simulink model "gm_combinedTxRx_AXIMM"  (R2017b)
settings: Solver=FixedStepDiscrete  StartTime=0.0  StopTime=10.0  RelTol=1e-3
InitFcn:
  | modelSettings
undefined symbols (not defined in the file or in its folder): coeff, filt, j, RadioSampleRate, VibertiTracebackLength, xPreambleSeq
libraries: hdlmdlgenlib x24, simulink x20, dsphdlfiltering x20, hdlsllib x10, dspsigops x5, commseqgen3 x4, commdigbbndpm3 x3, commcrc2 x2, commcnvcod2 x2, commsource2 x1, dspstat3 x1, dspmlti4 x1
(part 5 of 6)

== system gm_combinedTxRx_AXIMM/Combined TX and RX/Receiver HDL/Frame Recover/Gardner Timing Recovery/InterpControl_Blocks1/Calculate New mu ==
  note: Good at fixd(0,16,12)
  W : Inport  SampleTime=1e-06
  NCOCounter : Inport  Port=2  SampleTime=1e-06
  Math Reciprocal : Math  Operator=reciprocal  OutDataTypeStr=fixdt(1,16,12)  RndMeth=Zero  SaturateOnIntegerOverflow=on
  Product : Product  OutDataTypeStr=fixdt(0,15,14)
  mu : Outport  InitialOutput=0
  wires:
  W/1 -> Math Reciprocal/1
  NCOCounter/1 -> Product/2
  Math Reciprocal/1 -> Product/1
  Product/1 -> mu/1

== system gm_combinedTxRx_AXIMM/Combined TX and RX/Receiver HDL/Frame Recover/Gardner Timing Recovery/InterpControl_Blocks1/Mod 1 ==
  In1 : Inport  SampleTime=1e-06
  Add : Sum
  Compare To Constant : simulink/Logic and Bit Operations/Compare To Constant  relop=<  const=1  OutDataTypeStr=boolean
  Compare To Constant1 : simulink/Logic and Bit Operations/Compare To Constant  relop=>=  const=0  OutDataTypeStr=boolean
  Constant : Constant  OutDataTypeStr=fixdt(0,1,0)  SampleTime=-1
  Constant1 : Constant  OutDataTypeStr=fixdt(0,1,0)  SampleTime=-1
  Logical Operator : Logic  AllPortsSameDT=off  OutDataTypeStr=boolean
  Subtract : Sum  Inputs=+-
  Switch : Switch  Criteria=u2 > Threshold
  Switch1 : Switch
  Out1 : Outport  InitialOutput=0
  wires:
  In1/1 -> Switch1/2, Switch/1, Subtract/1, Compare To Constant1/1, Compare To Constant/1, Add/1
  Add/1 -> Switch1/3
  Compare To Constant/1 -> Logical Operator/2
  Compare To Constant1/1 -> Logical Operator/1
  Constant/1 -> Subtract/2
  Constant1/1 -> Add/2
  Logical Operator/1 -> Switch/2
  Subtract/1 -> Switch1/1
  Switch/1 -> Out1/1
  Switch1/1 -> Switch/3

== system gm_combinedTxRx_AXIMM/Combined TX and RX/Receiver HDL/Frame Recover/Gardner Timing Recovery/InterpControl_Blocks1/NCOCounter State ==
  in0 : Inport  OutDataTypeStr=fixdt(0, 16, 16)  SampleTime=1e-06
  Enable_out2 : EnablePort  OutDataTypeStr=boolean
  NCOCounter State : Delay  DelayLength=hex2num('3ff0000000000000')  InitialCondition=0  InputProcessing=Inherited
  out0 : Outport  OutDataTypeStr=fixdt(0, 16, 16)  InitialOutput=0
  wires:
  NCOCounter State/1 -> out0/1
  in0/1 -> NCOCounter State/1

== system gm_combinedTxRx_AXIMM/Combined TX and RX/Receiver HDL/Frame Recover/Gardner Timing Recovery/InterpControl_Blocks1/saved mu ==
  in0 : Inport  OutDataTypeStr=fixdt(0, 15, 14)  SampleTime=1e-06
  Enable_out2 : EnablePort  OutDataTypeStr=boolean
  saved mu : Delay  DelayLength=hex2num('3ff0000000000000')  InitialCondition=0  InputProcessing=Inherited
  out0 : Outport  OutDataTypeStr=fixdt(0, 15, 14)  InitialOutput=0
  wires:
  saved mu/1 -> out0/1
  in0/1 -> saved mu/1

== system gm_combinedTxRx_AXIMM/Combined TX and RX/Receiver HDL/Frame Recover/Gardner Timing Recovery/Interpolator/Delay ==
  in0 : Inport  OutDataTypeStr=fixdt(1, 16, 14)  SampleTime=1e-06
      settings: SignalType=complex
  Enable_out2 : EnablePort  OutDataTypeStr=boolean
  Delay : Delay  DelayLength=hex2num('3ff0000000000000')  InitialCondition=0  InputProcessing=Inherited
  out0 : Outport  OutDataTypeStr=fixdt(1, 16, 14)  InitialOutput=0
      settings: SignalType=complex
  wires:
  Delay/1 -> out0/1
  in0/1 -> Delay/1

== system gm_combinedTxRx_AXIMM/Combined TX and RX/Receiver HDL/Frame Recover/Gardner Timing Recovery/Interpolator/Delay1 ==
  in0 : Inport  OutDataTypeStr=fixdt(1, 16, 14)  SampleTime=1e-06
      settings: SignalType=complex
  Enable_out2 : EnablePort  OutDataTypeStr=boolean
  Delay1 : Delay  DelayLength=hex2num('3ff0000000000000')  InitialCondition=0  InputProcessing=Inherited
  out0 : Outport  OutDataTypeStr=fixdt(1, 16, 14)  InitialOutput=0
      settings: SignalType=complex
  wires:
  Delay1/1 -> out0/1
  in0/1 -> Delay1/1

== system gm_combinedTxRx_AXIMM/Combined TX and RX/Receiver HDL/Frame Recover/Gardner Timing Recovery/Interpolator/Delay2 ==
  in0 : Inport  OutDataTypeStr=fixdt(1, 16, 14)  SampleTime=1e-06
      settings: SignalType=complex
  Enable_out2 : EnablePort  OutDataTypeStr=boolean
  Delay2 : Delay  DelayLength=hex2num('3ff0000000000000')  InitialCondition=0  InputProcessing=Inherited
  out0 : Outport  OutDataTypeStr=fixdt(1, 16, 14)  InitialOutput=0
      settings: SignalType=complex
  wires:
  Delay2/1 -> out0/1
  in0/1 -> Delay2/1

== system gm_combinedTxRx_AXIMM/Combined TX and RX/Receiver HDL/Frame Recover/Gardner Timing Recovery/Interpolator/Delay3 ==
  in0 : Inport  OutDataTypeStr=fixdt(1, 16, 13)  SampleTime=1e-06
      settings: SignalType=complex
  Enable_out2 : EnablePort  OutDataTypeStr=boolean
  Delay3 : Delay  DelayLength=hex2num('3ff0000000000000')  InitialCondition=0  InputProcessing=Inherited
  out0 : Outport  OutDataTypeStr=fixdt(1, 16, 13)  InitialOutput=0
      settings: SignalType=complex
  wires:
  Delay3/1 -> out0/1
  in0/1 -> Delay3/1

== system gm_combinedTxRx_AXIMM/Combined TX and RX/Receiver HDL/Frame Recover/Gardner Timing Recovery/Interpolator/Delay4 ==
  in0 : Inport  OutDataTypeStr=fixdt(1, 16, 13)  SampleTime=1e-06
      settings: SignalType=complex
  Enable_out2 : EnablePort  OutDataTypeStr=boolean
  Delay4 : Delay  DelayLength=hex2num('3ff0000000000000')  InitialCondition=0  InputProcessing=Inherited
  out0 : Outport  OutDataTypeStr=fixdt(1, 16, 13)  InitialOutput=0
      settings: SignalType=complex
  wires:
  Delay4/1 -> out0/1
  in0/1 -> Delay4/1

== system gm_combinedTxRx_AXIMM/Combined TX and RX/Receiver HDL/Frame Recover/Gardner Timing Recovery/Interpolator/PLD ==
  in0 : Inport  OutDataTypeStr=fixdt(1, 20, 14)  SampleTime=1e-06
      settings: SignalType=complex
  Enable_out2 : EnablePort  OutDataTypeStr=boolean
  PLD : Delay  DelayLength=hex2num('3ff0000000000000')  InitialCondition=0  InputProcessing=Inherited
  out0 : Outport  OutDataTypeStr=fixdt(1, 20, 14)  InitialOutput=0
      settings: SignalType=complex
  wires:
  PLD/1 -> out0/1
  in0/1 -> PLD/1

== system gm_combinedTxRx_AXIMM/Combined TX and RX/Receiver HDL/Frame Recover/Gardner Timing Recovery/Interpolator/PLD1 ==
  in0 : Inport  OutDataTypeStr=fixdt(1, 18, 14)  SampleTime=1e-06
      settings: SignalType=complex
  Enable_out2 : EnablePort  OutDataTypeStr=boolean
  PLD1 : Delay  DelayLength=hex2num('3ff0000000000000')  InitialCondition=0  InputProcessing=Inherited
  out0 : Outport  OutDataTypeStr=fixdt(1, 18, 14)  InitialOutput=0
      settings: SignalType=complex
  wires:
  PLD1/1 -> out0/1
  in0/1 -> PLD1/1

== system gm_combinedTxRx_AXIMM/Combined TX and RX/Receiver HDL/Frame Recover/Gardner Timing Recovery/Interpolator/PLD2 ==
  in0 : Inport  OutDataTypeStr=fixdt(0, 15, 14)  SampleTime=1e-06
  Enable_out2 : EnablePort  OutDataTypeStr=boolean
  PLD2 : Delay  DelayLength=hex2num('3ff0000000000000')  InitialCondition=0  InputProcessing=Inherited
  out0 : Outport  OutDataTypeStr=fixdt(0, 15, 14)  InitialOutput=0
  wires:
  PLD2/1 -> out0/1
  in0/1 -> PLD2/1

== system gm_combinedTxRx_AXIMM/Combined TX and RX/Receiver HDL/Frame Recover/Gardner Timing Recovery/Interpolator/PLD3 ==
  in0 : Inport  OutDataTypeStr=fixdt(1, 16, 13)  SampleTime=1e-06
      settings: SignalType=complex
  Enable_out2 : EnablePort  OutDataTypeStr=boolean
  PLD3 : Delay  DelayLength=hex2num('3ff0000000000000')  InitialCondition=0  InputProcessing=Inherited
  out0 : Outport  OutDataTypeStr=fixdt(1, 16, 13)  InitialOutput=0
      settings: SignalType=complex
  wires:
  PLD3/1 -> out0/1
  in0/1 -> PLD3/1

== system gm_combinedTxRx_AXIMM/Combined TX and RX/Receiver HDL/Frame Recover/Gardner Timing Recovery/Interpolator/PLD4 ==
  in0 : Inport  OutDataTypeStr=fixdt(1, 16, 13)  SampleTime=1e-06
      settings: SignalType=complex
  Enable_out2 : EnablePort  OutDataTypeStr=boolean
  PLD4 : Delay  DelayLength=hex2num('3ff0000000000000')  InitialCondition=0  InputProcessing=Inherited
  out0 : Outport  OutDataTypeStr=fixdt(1, 16, 13)  InitialOutput=0
      settings: SignalType=complex
  wires:
  PLD4/1 -> out0/1
  in0/1 -> PLD4/1

== system gm_combinedTxRx_AXIMM/Combined TX and RX/Receiver HDL/Frame Recover/Gardner Timing Recovery/Interpolator/PLD5 ==
  in0 : Inport  OutDataTypeStr=fixdt(1, 21, 14)  SampleTime=1e-06
      settings: SignalType=complex
  Enable_out2 : EnablePort  OutDataTypeStr=boolean
  PLD5 : Delay  DelayLength=hex2num('3ff0000000000000')  InitialCondition=0  InputProcessing=Inherited
  out0 : Outport  OutDataTypeStr=fixdt(1, 21, 14)  InitialOutput=0
      settings: SignalType=complex
  wires:
  PLD5/1 -> out0/1
  in0/1 -> PLD5/1

== system gm_combinedTxRx_AXIMM/Combined TX and RX/Receiver HDL/Frame Recover/Gardner Timing Recovery/Interpolator/PLD6 ==
  in0 : Inport  OutDataTypeStr=fixdt(0, 15, 14)  SampleTime=1e-06
  Enable_out2 : EnablePort  OutDataTypeStr=boolean
  PLD6 : Delay  DelayLength=hex2num('3ff0000000000000')  InitialCondition=0  InputProcessing=Inherited
  out0 : Outport  OutDataTypeStr=fixdt(0, 15, 14)  InitialOutput=0
  wires:
  PLD6/1 -> out0/1
  in0/1 -> PLD6/1

== system gm_combinedTxRx_AXIMM/Combined TX and RX/Receiver HDL/Frame Recover/Gardner Timing Recovery/Interpolator/PLD7 ==
  in0 : Inport  OutDataTypeStr=fixdt(1, 16, 10)  SampleTime=1e-06
      settings: SignalType=complex
  Enable_out2 : EnablePort  OutDataTypeStr=boolean
  PLD7 : Delay  DelayLength=hex2num('4000000000000000')  InitialCondition=0  InputProcessing=Inherited
  out0 : Outport  OutDataTypeStr=fixdt(1, 16, 10)  InitialOutput=0
      settings: SignalType=complex
  wires:
  PLD7/1 -> out0/1
  in0/1 -> PLD7/1

== system gm_combinedTxRx_AXIMM/Combined TX and RX/Receiver HDL/Frame Recover/Gardner Timing Recovery/LoopFilter1/Delay1 ==
  in0 : Inport  OutDataTypeStr=fixdt(1, 16, 24)  SampleTime=1e-06
  Enable_out2 : EnablePort  OutDataTypeStr=boolean
  Delay1 : Delay  DelayLength=hex2num('3ff0000000000000')  InitialCondition=0  InputProcessing=Inherited
  out0 : Outport  OutDataTypeStr=fixdt(1, 16, 24)  InitialOutput=0
  wires:
  Delay1/1 -> out0/1
  in0/1 -> Delay1/1

== system gm_combinedTxRx_AXIMM/Combined TX and RX/Receiver HDL/Frame Recover/Gardner Timing Recovery/LoopFilter1/Delay2 ==
  in0 : Inport  OutDataTypeStr=fixdt(1, 16, 15)  SampleTime=1e-06
  Enable_out2 : EnablePort  OutDataTypeStr=boolean
  Delay2 : Delay  DelayLength=hex2num('3ff0000000000000')  InitialCondition=0  InputProcessing=Inherited
  out0 : Outport  OutDataTypeStr=fixdt(1, 16, 15)  InitialOutput=0
  wires:
  Delay2/1 -> out0/1
  in0/1 -> Delay2/1

== system gm_combinedTxRx_AXIMM/Combined TX and RX/Receiver HDL/Frame Recover/Gardner Timing Recovery/TED Lock Detector/MATLAB Function ==
  u : Inport  SampleTime=1e-06
  RxTxFixedPointLibrary_c5_MATLAB_Function : MATLAB Function  TreatAsAtomicUnit=on
  y : Outport  InitialOutput=0
  wires:
  RxTxFixedPointLibrary_c5_MATLAB_Function/1(y) -> y/1
  u/1 -> RxTxFixedPointLibrary_c5_MATLAB_Function/1(u)

== system gm_combinedTxRx_AXIMM/Combined TX and RX/Receiver HDL/Frame Recover/Gardner Timing Recovery/TED Lock Detector/Pipeline Delay ==
  in0 : Inport  OutDataTypeStr=fixdt(1, 16, 15)  SampleTime=1e-06
  Enable_out2 : EnablePort  OutDataTypeStr=boolean
  Pipeline Delay : Delay  DelayLength=hex2num('3ff0000000000000')  InitialCondition=0  InputProcessing=Inherited
  out0 : Outport  OutDataTypeStr=fixdt(1, 16, 15)  InitialOutput=0
  wires:
  Pipeline Delay/1 -> out0/1
  in0/1 -> Pipeline Delay/1

== system gm_combinedTxRx_AXIMM/Combined TX and RX/Receiver HDL/Frame Recover/Gardner Timing Recovery/TED Lock Detector/Tapped Delay ==
  in0 : Inport  OutDataTypeStr=fixdt(0, 16, 15)  SampleTime=1e-06
  Enable_out2 : EnablePort  OutDataTypeStr=boolean
  Tapped Delay : simulink/Discrete/Tapped Delay  vinit=0  samptime=-1  NumDelays=hex2num('4059000000000000')  DelayOrder=Oldest  includeCurrent=off
  out0 : Outport  OutDataTypeStr=fixdt(0, 16, 15)  PortDimensions=[100]  InitialOutput=0
  wires:
  Tapped Delay/1 -> out0/1
  in0/1 -> Tapped Delay/1

== system gm_combinedTxRx_AXIMM/Combined TX and RX/Transmitter HDL/Packet Generation/Payload/HDL Scrambler 2 bits/Buffer Manage ==
  bit1 : Inport  SampleTime=4e-06
  bit2 : Inport  Port=2  SampleTime=4e-06
  reset : Inport  Port=3  SampleTime=4e-06
  RxTxFixedPointLibrary_c20_Buffer_Manage : MATLAB Function  TreatAsAtomicUnit=on
  outBuffer : Outport
  wires:
  bit1/1 -> RxTxFixedPointLibrary_c20_Buffer_Manage/1(bit1)
  bit2/1 -> RxTxFixedPointLibrary_c20_Buffer_Manage/2(bit2)
  reset/1 -> RxTxFixedPointLibrary_c20_Buffer_Manage/3(reset)
  RxTxFixedPointLibrary_c20_Buffer_Manage/1(outBuffer) -> outBuffer/1

== system gm_combinedTxRx_AXIMM/Combined TX and RX/Transmitter HDL/Packet Generation/Payload/Subsystem/MATLAB Function3 ==
  start : Inport  SampleTime=4e-06
  done : Inport  Port=2  SampleTime=4e-06
  RxTxFixedPointLibrary_c9_MATLAB_Function3 : MATLAB Function  TreatAsAtomicUnit=on
  enable : Outport
  wires:
  start/1 -> RxTxFixedPointLibrary_c9_MATLAB_Function3/1(start)
  done/1 -> RxTxFixedPointLibrary_c9_MATLAB_Function3/2(done)
  RxTxFixedPointLibrary_c9_MATLAB_Function3/1(enable) -> enable/1

== system gm_combinedTxRx_AXIMM/Combined TX and RX/Receiver HDL/Frame Recover/Equalization and Demodulation/2 Bit Descrambler/MATLAB Function/MATLAB Function ==
  bits : Inport  PortDimensions=2  SampleTime=1e-06
  reset : Inport  Port=2  SampleTime=1e-06
  RxTxFixedPointLibrary_c10_MATLAB_Function : MATLAB Function  TreatAsAtomicUnit=on
  bufferA : Outport  InitialOutput=0
  bufferB : Outport  Port=2  InitialOutput=0
  wires:
  bits/1 -> RxTxFixedPointLibrary_c10_MATLAB_Function/1(bits)
  reset/1 -> RxTxFixedPointLibrary_c10_MATLAB_Function/2(reset)
  RxTxFixedPointLibrary_c10_MATLAB_Function/1(bufferA) -> bufferA/1
  RxTxFixedPointLibrary_c10_MATLAB_Function/2(bufferB) -> bufferB/1

== system gm_combinedTxRx_AXIMM/Combined TX and RX/Receiver HDL/Frame Recover/Equalization and Demodulation/DFE/DFE/Backward Taps ==
  in0 : Inport  OutDataTypeStr=fixdt(1, 16, 15)  PortDimensions=[3]  SampleTime=1e-06
      settings: SignalType=complex
  Enable_out4 : EnablePort  OutDataTypeStr=boolean
  Backward Taps : UnitDelay  InitialCondition="[0  0  0]"  SampleTime=1e-06
  out0 : Outport  OutDataTypeStr=fixdt(1, 16, 15)  PortDimensions=[3]  InitialOutput=0
      settings: SignalType=complex
  wires:
  Backward Taps/1 -> out0/1
  in0/1 -> Backward Taps/1

== system gm_combinedTxRx_AXIMM/Combined TX and RX/Receiver HDL/Frame Recover/Equalization and Demodulation/DFE/DFE/Decision Buffer_tap0 ==
  in0 : Inport  OutDataTypeStr=fixdt(1, 16, 15)  SampleTime=1e-06
      settings: SignalType=complex
  Enable_out4 : EnablePort  OutDataTypeStr=boolean
  Decision Buffer_tap0 : Delay  DelayLength=hex2num('3ff0000000000000')  InputProcessing=Inherited
  out0 : Outport  OutDataTypeStr=fixdt(1, 16, 15)  InitialOutput=0
      settings: SignalType=complex
  wires:
  Decision Buffer_tap0/1 -> out0/1
  in0/1 -> Decision Buffer_tap0/1

== system gm_combinedTxRx_AXIMM/Combined TX and RX/Receiver HDL/Frame Recover/Equalization and Demodulation/DFE/DFE/Decision Buffer_tap1 ==
  in0 : Inport  OutDataTypeStr=fixdt(1, 16, 15)  SampleTime=1e-06
      settings: SignalType=complex
  Enable_out4 : EnablePort  OutDataTypeStr=boolean
  Decision Buffer_tap1 : Delay  DelayLength=hex2num('3ff0000000000000')  InputProcessing=Inherited
  out0 : Outport  OutDataTypeStr=fixdt(1, 16, 15)  InitialOutput=0
      settings: SignalType=complex
  wires:
  Decision Buffer_tap1/1 -> out0/1
  in0/1 -> Decision Buffer_tap1/1

== system gm_combinedTxRx_AXIMM/Combined TX and RX/Receiver HDL/Frame Recover/Equalization and Demodulation/DFE/DFE/Decision Buffer_tap2 ==
  in0 : Inport  OutDataTypeStr=fixdt(1, 16, 15)  SampleTime=1e-06
      settings: SignalType=complex
  Enable_out4 : EnablePort  OutDataTypeStr=boolean
  Decision Buffer_tap2 : Delay  DelayLength=hex2num('3ff0000000000000')  InputProcessing=Inherited
  out0 : Outport  OutDataTypeStr=fixdt(1, 16, 15)  InitialOutput=0
      settings: SignalType=complex
  wires:
  Decision Buffer_tap2/1 -> out0/1
  in0/1 -> Decision Buffer_tap2/1

== system gm_combinedTxRx_AXIMM/Combined TX and RX/Receiver HDL/Frame Recover/Equalization and Demodulation/DFE/DFE/Delay To Reference Tap2 ==
  in0 : Inport  OutDataTypeStr=boolean  SampleTime=1e-06
  Enable_out4 : EnablePort  OutDataTypeStr=boolean
  Delay To Reference Tap2 : Delay  DelayLength=hex2num('4008000000000000')  InitialCondition=0  InputProcessing=Inherited
  out0 : Outport  OutDataTypeStr=boolean  InitialOutput=0
  wires:
  Delay To Reference Tap2/1 -> out0/1
  in0/1 -> Delay To Reference Tap2/1

== system gm_combinedTxRx_AXIMM/Combined TX and RX/Receiver HDL/Frame Recover/Equalization and Demodulation/DFE/DFE/Delay To Reference Tap_lowered ==
  in0 : Inport  OutDataTypeStr=fixdt(1, 16, 15)  SampleTime=1e-06
      settings: SignalType=complex
  Enable_out4 : EnablePort  OutDataTypeStr=boolean
  Delay To Reference Tap_lowered : Delay  DelayLength=hex2num('3ff0000000000000')  InitialCondition=0  InputProcessing=Inherited
  out0 : Outport  OutDataTypeStr=fixdt(1, 16, 15)  InitialOutput=0
      settings: SignalType=complex
  wires:
  Delay To Reference Tap_lowered/1 -> out0/1
  in0/1 -> Delay To Reference Tap_lowered/1

== system gm_combinedTxRx_AXIMM/Combined TX and RX/Receiver HDL/Frame Recover/Equalization and Demodulation/DFE/DFE/Delay To Reference Tap_lowered1 ==
  in0 : Inport  OutDataTypeStr=fixdt(1, 16, 15)  SampleTime=1e-06
      settings: SignalType=complex
  Enable_out4 : EnablePort  OutDataTypeStr=boolean
  Delay To Reference Tap_lowered : Delay  DelayLength=hex2num('3ff0000000000000')  InitialCondition=0  InputProcessing=Inherited
  out0 : Outport  OutDataTypeStr=fixdt(1, 16, 15)  InitialOutput=0
      settings: SignalType=complex
  wires:
  Delay To Reference Tap_lowered/1 -> out0/1
  in0/1 -> Delay To Reference Tap_lowered/1

== system gm_combinedTxRx_AXIMM/Combined TX and RX/Receiver HDL/Frame Recover/Equalization and Demodulation/DFE/DFE/Delay data so DFE can reset1 ==
  in0 : Inport  OutDataTypeStr=boolean  SampleTime=1e-06
  Enable_out4 : EnablePort  OutDataTypeStr=boolean
  Delay data so DFE can reset1 : Delay  DelayLength=hex2num('3ff0000000000000')  InitialCondition=0  InputProcessing=Inherited
  out0 : Outport  OutDataTypeStr=boolean  InitialOutput=0
  wires:
  Delay data so DFE can reset1/1 -> out0/1
  in0/1 -> Delay data so DFE can reset1/1

== system gm_combinedTxRx_AXIMM/Combined TX and RX/Receiver HDL/Frame Recover/Equalization and Demodulation/DFE/DFE/Forward Taps ==
  in0 : Inport  OutDataTypeStr=fixdt(1, 16, 14)  PortDimensions=[5]  SampleTime=1e-06
      settings: SignalType=complex
  Enable_out4 : EnablePort  OutDataTypeStr=boolean
  Forward Taps : UnitDelay  InitialCondition=hex2num('0000000000000000')  SampleTime=1e-06
  out0 : Outport  OutDataTypeStr=fixdt(1, 16, 14)  PortDimensions=[5]  InitialOutput=0
      settings: SignalType=complex
  wires:
  Forward Taps/1 -> out0/1
  in0/1 -> Forward Taps/1

== system gm_combinedTxRx_AXIMM/Combined TX and RX/Receiver HDL/Frame Recover/Equalization and Demodulation/DFE/DFE/Forward Taps_ctrl_delay ==
  in0 : Inport  OutDataTypeStr=boolean  SampleTime=1e-06
  Enable_out4 : EnablePort  OutDataTypeStr=boolean
  Forward Taps_ctrl_delay : Delay  DelayLength=hex2num('3ff0000000000000')  InitialCondition=0  InputProcessing=Inherited
  out0 : Outport  OutDataTypeStr=boolean  InitialOutput=0
  wires:
  Forward Taps_ctrl_delay/1 -> out0/1
  in0/1 -> Forward Taps_ctrl_delay/1

== system gm_combinedTxRx_AXIMM/Combined TX and RX/Receiver HDL/Frame Recover/Equalization and Demodulation/DFE/DFE/InputBuffer_tap0 ==
  in0 : Inport  OutDataTypeStr=fixdt(1, 16, 14)  SampleTime=1e-06
      settings: SignalType=complex
  Enable_out4 : EnablePort  OutDataTypeStr=boolean
  InputBuffer_tap0 : Delay  DelayLength=hex2num('3ff0000000000000')  InputProcessing=Inherited
  out0 : Outport  OutDataTypeStr=fixdt(1, 16, 14)  InitialOutput=0
      settings: SignalType=complex
  wires:
  InputBuffer_tap0/1 -> out0/1
  in0/1 -> InputBuffer_tap0/1

== system gm_combinedTxRx_AXIMM/Combined TX and RX/Receiver HDL/Frame Recover/Equalization and Demodulation/DFE/DFE/InputBuffer_tap1 ==
  in0 : Inport  OutDataTypeStr=fixdt(1, 16, 14)  SampleTime=1e-06
      settings: SignalType=complex
  Enable_out4 : EnablePort  OutDataTypeStr=boolean
  InputBuffer_tap1 : Delay  DelayLength=hex2num('3ff0000000000000')  InputProcessing=Inherited
  out0 : Outport  OutDataTypeStr=fixdt(1, 16, 14)  InitialOutput=0
      settings: SignalType=complex
  wires:
  InputBuffer_tap1/1 -> out0/1
  in0/1 -> InputBuffer_tap1/1

== system gm_combinedTxRx_AXIMM/Combined TX and RX/Receiver HDL/Frame Recover/Equalization and Demodulation/DFE/DFE/InputBuffer_tap2 ==
  in0 : Inport  OutDataTypeStr=fixdt(1, 16, 14)  SampleTime=1e-06
      settings: SignalType=complex
  Enable_out4 : EnablePort  OutDataTypeStr=boolean
  InputBuffer_tap2 : Delay  DelayLength=hex2num('3ff0000000000000')  InputProcessing=Inherited
  out0 : Outport  OutDataTypeStr=fixdt(1, 16, 14)  InitialOutput=0
      settings: SignalType=complex
  wires:
  InputBuffer_tap2/1 -> out0/1
  in0/1 -> InputBuffer_tap2/1

== system gm_combinedTxRx_AXIMM/Combined TX and RX/Receiver HDL/Frame Recover/Equalization and Demodulation/DFE/DFE/InputBuffer_tap3 ==
  in0 : Inport  OutDataTypeStr=fixdt(1, 16, 14)  SampleTime=1e-06
      settings: SignalType=complex
  Enable_out4 : EnablePort  OutDataTypeStr=boolean
  InputBuffer_tap3 : Delay  DelayLength=hex2num('3ff0000000000000')  InputProcessing=Inherited
  out0 : Outport  OutDataTypeStr=fixdt(1, 16, 14)  InitialOutput=0
      settings: SignalType=complex
  wires:
  InputBuffer_tap3/1 -> out0/1
  in0/1 -> InputBuffer_tap3/1

== system gm_combinedTxRx_AXIMM/Combined TX and RX/Receiver HDL/Frame Recover/Equalization and Demodulation/DFE/DFE/InputBuffer_tap4 ==
  in0 : Inport  OutDataTypeStr=fixdt(1, 16, 14)  SampleTime=1e-06
      settings: SignalType=complex
  Enable_out4 : EnablePort  OutDataTypeStr=boolean
  InputBuffer_tap4 : Delay  DelayLength=hex2num('3ff0000000000000')  InputProcessing=Inherited
  out0 : Outport  OutDataTypeStr=fixdt(1, 16, 14)  InitialOutput=0
      settings: SignalType=complex
  wires:
  InputBuffer_tap4/1 -> out0/1
  in0/1 -> InputBuffer_tap4/1

== system gm_combinedTxRx_AXIMM/Combined TX and RX/Receiver HDL/Frame Recover/Equalization and Demodulation/DFE/DFE/Map Symbol ==
  In1 : Inport  OutDataTypeStr=fixdt(1,16,14)  SampleTime=1e-06
  training : Inport  Port=2  OutDataTypeStr=fixdt(1,16,15)  SampleTime=1e-06
  reset : Inport  Port=3  SampleTime=1e-06
  Enable_out4 : Inport  Port=4  OutDataTypeStr=boolean  SampleTime=1e-06
  Decision Directed : Subsystem
  Delay : Subsystem
      settings: MinAlgLoopOccurrences=on
  HDL Counter : Subsystem
      settings: MinAlgLoopOccurrences=on
  Switch : Switch  Criteria=u2 > Threshold  Threshold=hex2num('406f400000000000')  OutDataTypeStr=fixdt(1, 16, 15)  SampleTime=1e-06
  d : Outport  InitialOutput=0
  wires:
  In1/1 -> Decision Directed/1(eqOut)
  training/1 -> Delay/1(in0)
  reset/1 -> HDL Counter/1(in0)
  Decision Directed/1(decision) -> Switch/1
  Delay/1(out0) -> Switch/3
  HDL Counter/1(out0) -> Switch/2
  Switch/1 -> d/1
  Enable_out4/1 -> HDL Counter/Enable, Delay/Enable

== system gm_combinedTxRx_AXIMM/Combined TX and RX/Receiver HDL/Frame Recover/Equalization and Demodulation/DFE/DFE/Pipeline Delay1 ==
  in0 : Inport  OutDataTypeStr=int16  SampleTime=1e-06
  Enable_out4 : EnablePort  OutDataTypeStr=boolean
  Pipeline Delay1 : Delay  DelayLength=hex2num('3ff0000000000000')  InitialCondition=0  InputProcessing=Inherited
  out0 : Outport  OutDataTypeStr=int16  InitialOutput=0
  wires:
  Pipeline Delay1/1 -> out0/1
  in0/1 -> Pipeline Delay1/1

== system gm_combinedTxRx_AXIMM/Combined TX and RX/Receiver HDL/Frame Recover/Equalization and Demodulation/DFE/DFE/Pipeline Delay2 ==
  in0 : Inport  OutDataTypeStr=fixdt(0, 16, 22)  SampleTime=1e-06
  Enable_out4 : EnablePort  OutDataTypeStr=boolean
  Pipeline Delay2 : Delay  DelayLength=hex2num('3ff0000000000000')  InitialCondition=0  InputProcessing=Inherited
  out0 : Outport  OutDataTypeStr=fixdt(0, 16, 22)  InitialOutput=0
  wires:
  Pipeline Delay2/1 -> out0/1
  in0/1 -> Pipeline Delay2/1

== system gm_combinedTxRx_AXIMM/Combined TX and RX/Receiver HDL/Frame Recover/Gardner Timing Recovery/Gardner TED Blocks/Imag Error/Delay ==
  in0 : Inport  OutDataTypeStr=fixdt(1, 16, 10)  SampleTime=1e-06
  Enable_out2 : EnablePort  OutDataTypeStr=boolean
  Delay : Delay  DelayLength=hex2num('3ff0000000000000')  InitialCondition=0  InputProcessing=Inherited
  out0 : Outport  OutDataTypeStr=fixdt(1, 16, 10)  InitialOutput=0
  wires:
  Delay/1 -> out0/1
  in0/1 -> Delay/1

== system gm_combinedTxRx_AXIMM/Combined TX and RX/Receiver HDL/Frame Recover/Gardner Timing Recovery/Gardner TED Blocks/Imag Error/TED Buffer Update1 ==
  new data : Inport  SampleTime=1e-06
  strobe sum : Inport  Port=2  SampleTime=1e-06
  Enable_out2 : Inport  Port=3  OutDataTypeStr=boolean  SampleTime=1e-06
  Delay : Subsystem
      settings: MinAlgLoopOccurrences=on
  Delay1 : Subsystem
      settings: MinAlgLoopOccurrences=on
  Delay2 : Subsystem
      settings: MinAlgLoopOccurrences=on
  Delay3 : Subsystem
      settings: MinAlgLoopOccurrences=on
  Multiport Switch{,1..3} (4 alike) : MultiPortSwitch  DataPortOrder=Zero-based contiguous  DiagnosticForDefault=None  OutDataTypeStr=fixdt(1, 16, 10)  SampleTime=1e-06
  Zero bit : Constant  Value=fi(0,1,16,13,'hex','0000')  OutDataTypeStr=fixdt(1, 16, 13)  SampleTime=-1
  Middle Indx : Outport  InitialOutput=0
  oldest : Outport  Port=2  InitialOutput=0
  wires:
  new data/1 -> Multiport Switch3/4, Multiport Switch3/3
  strobe sum/1 -> Multiport Switch3/1, Multiport Switch2/1, Multiport Switch1/1, Multiport Switch/1
  Delay/1(out0) -> Multiport Switch/2
  Delay1/1(out0) -> Multiport Switch1/2, Multiport Switch/3
  Delay2/1(out0) -> Multiport Switch2/2, Multiport Switch1/3, Multiport Switch/4
  Delay3/1(out0) -> Multiport Switch3/2, Multiport Switch2/3, Multiport Switch1/4
  Multiport Switch/1 -> Delay/1(in0), oldest/1
  Multiport Switch1/1 -> Delay1/1(in0)
  Multiport Switch2/1 -> Delay2/1(in0), Middle Indx/1
  Multiport Switch3/1 -> Delay3/1(in0)
  Zero bit/1 -> Multiport Switch2/4
  Enable_out2/1 -> Delay3/Enable, Delay2/Enable, Delay1/Enable, Delay/Enable

== system gm_combinedTxRx_AXIMM/Combined TX and RX/Receiver HDL/Frame Recover/Gardner Timing Recovery/Gardner TED Blocks/Real Error/Delay ==
  in0 : Inport  OutDataTypeStr=fixdt(1, 16, 10)  SampleTime=1e-06
  Enable_out2 : EnablePort  OutDataTypeStr=boolean
  Delay : Delay  DelayLength=hex2num('3ff0000000000000')  InitialCondition=0  InputProcessing=Inherited
  out0 : Outport  OutDataTypeStr=fixdt(1, 16, 10)  InitialOutput=0
  wires:
  Delay/1 -> out0/1
  in0/1 -> Delay/1

== system gm_combinedTxRx_AXIMM/Combined TX and RX/Receiver HDL/Frame Recover/Gardner Timing Recovery/Gardner TED Blocks/Real Error/TED Buffer Update1 ==
  new data : Inport  SampleTime=1e-06
  strobe sum : Inport  Port=2  SampleTime=1e-06
  Enable_out2 : Inport  Port=3  OutDataTypeStr=boolean  SampleTime=1e-06
  Delay : Subsystem
      settings: MinAlgLoopOccurrences=on
  Delay1 : Subsystem
      settings: MinAlgLoopOccurrences=on
  Delay2 : Subsystem
      settings: MinAlgLoopOccurrences=on
  Delay3 : Subsystem
      settings: MinAlgLoopOccurrences=on
  Multiport Switch{,1..3} (4 alike) : MultiPortSwitch  DataPortOrder=Zero-based contiguous  DiagnosticForDefault=None  OutDataTypeStr=fixdt(1, 16, 10)  SampleTime=1e-06
  Zero bit : Constant  Value=fi(0,1,16,13,'hex','0000')  OutDataTypeStr=fixdt(1, 16, 13)  SampleTime=-1
  Middle Indx : Outport  InitialOutput=0
  oldest : Outport  Port=2  InitialOutput=0
  wires:
  new data/1 -> Multiport Switch3/4, Multiport Switch3/3
  strobe sum/1 -> Multiport Switch3/1, Multiport Switch2/1, Multiport Switch1/1, Multiport Switch/1
  Delay/1(out0) -> Multiport Switch/2
  Delay1/1(out0) -> Multiport Switch1/2, Multiport Switch/3
  Delay2/1(out0) -> Multiport Switch2/2, Multiport Switch1/3, Multiport Switch/4
  Delay3/1(out0) -> Multiport Switch3/2, Multiport Switch2/3, Multiport Switch1/4
  Multiport Switch/1 -> Delay/1(in0), oldest/1
  Multiport Switch1/1 -> Delay1/1(in0)
  Multiport Switch2/1 -> Delay2/1(in0), Middle Indx/1
  Multiport Switch3/1 -> Delay3/1(in0)
  Zero bit/1 -> Multiport Switch2/4
  Enable_out2/1 -> Delay3/Enable, Delay2/Enable, Delay1/Enable, Delay/Enable

== system gm_combinedTxRx_AXIMM/Combined TX and RX/Receiver HDL/Frame Recover/Equalization and Demodulation/DFE/DFE/Map Symbol/Decision Directed ==
  eqOut : Inport  OutDataTypeStr=fixdt(1,16,14)  SampleTime=1e-06
  Compare To Zero : simulink/Logic and Bit Operations/Compare To Constant  relop=>=  const=hex2num('0000000000000000')  OutDataTypeStr=boolean
  Compare To Zero1 : simulink/Logic and Bit Operations/Compare To Constant  relop=>=  const=hex2num('0000000000000000')  OutDataTypeStr=boolean
  Complex to Real-Imag : ComplexToRealImag  SampleTime=1e-06
  QPSK Decisions : LookupNDDirect  Table="reshape([complex(-0.7071, -0.7071) complex(0.7071, -0.7071) complex(-0.7071, 0.7071) complex(0.7071, 0.7071)].', [2  2])"  DiagnosticForOutOfRangeInput=Error  SampleTime=1e-06  TableDataTypeStr=fixdt(1,16,15)
  decision : Outport  InitialOutput=0
  wires:
  eqOut/1 -> Complex to Real-Imag/1
  Compare To Zero/1 -> QPSK Decisions/1
  Compare To Zero1/1 -> QPSK Decisions/2
  Complex to Real-Imag/1 -> Compare To Zero/1
  Complex to Real-Imag/2 -> Compare To Zero1/1
  QPSK Decisions/1 -> decision/1

== system gm_combinedTxRx_AXIMM/Combined TX and RX/Receiver HDL/Frame Recover/Equalization and Demodulation/DFE/DFE/Map Symbol/Delay ==
  in0 : Inport  OutDataTypeStr=fixdt(1, 16, 15)  SampleTime=1e-06
      settings: SignalType=complex
  Enable_out4 : EnablePort  OutDataTypeStr=boolean
  Delay : Delay  DelayLength=hex2num('3ff0000000000000')  InitialCondition=0  InputProcessing=Inherited
  out0 : Outport  OutDataTypeStr=fixdt(1, 16, 15)  InitialOutput=0
      settings: SignalType=complex
  wires:
  Delay/1 -> out0/1
  in0/1 -> Delay/1

== system gm_combinedTxRx_AXIMM/Combined TX and RX/Receiver HDL/Frame Recover/Equalization and Demodulation/DFE/DFE/Map Symbol/HDL Counter ==
  in0 : Inport  OutDataTypeStr=boolean  SampleTime=1e-06
  Enable_out4 : EnablePort  OutDataTypeStr=boolean
  HDL Counter : hdlsllib/Sources/HDL Counter  CountType=Count limited  CountInit=hex2num('0000000000000000')  CountStep=hex2num('3ff0000000000000')  CountMax=hex2num('4110000000000000')  CountFromType=Initial value  CountFrom=hex2num('0000000000000000')  CountResetPort=on  CountLoadPort=off  CountEnbPort=off  CountDirPort=off  CountDataType=Unsigned  CountWordLen=32  CountFracLen=0  CountSampTime=1e-06
      settings: SourceProductBaseCode=HD
  out0 : Outport  OutDataTypeStr=uint32  InitialOutput=0
  wires:
  HDL Counter/1 -> out0/1
  in0/1 -> HDL Counter/1

== system gm_combinedTxRx_AXIMM/Combined TX and RX/Receiver HDL/Frame Recover/Gardner Timing Recovery/Gardner TED Blocks/Imag Error/TED Buffer Update1/Delay ==
  in0 : Inport  OutDataTypeStr=fixdt(1, 16, 10)  SampleTime=1e-06
  Enable_out2 : EnablePort  OutDataTypeStr=boolean
  Delay : Delay  DelayLength=hex2num('3ff0000000000000')  InitialCondition=0  InputProcessing=Inherited
  out0 : Outport  OutDataTypeStr=fixdt(1, 16, 10)  InitialOutput=0
  wires:
  Delay/1 -> out0/1
  in0/1 -> Delay/1

== system gm_combinedTxRx_AXIMM/Combined TX and RX/Receiver HDL/Frame Recover/Gardner Timing Recovery/Gardner TED Blocks/Imag Error/TED Buffer Update1/Delay1 ==
  in0 : Inport  OutDataTypeStr=fixdt(1, 16, 10)  SampleTime=1e-06
  Enable_out2 : EnablePort  OutDataTypeStr=boolean
  Delay1 : Delay  DelayLength=hex2num('3ff0000000000000')  InitialCondition=0  InputProcessing=Inherited
  out0 : Outport  OutDataTypeStr=fixdt(1, 16, 10)  InitialOutput=0
  wires:
  Delay1/1 -> out0/1
  in0/1 -> Delay1/1

== system gm_combinedTxRx_AXIMM/Combined TX and RX/Receiver HDL/Frame Recover/Gardner Timing Recovery/Gardner TED Blocks/Imag Error/TED Buffer Update1/Delay2 ==
  in0 : Inport  OutDataTypeStr=fixdt(1, 16, 10)  SampleTime=1e-06
  Enable_out2 : EnablePort  OutDataTypeStr=boolean
  Delay2 : Delay  DelayLength=hex2num('3ff0000000000000')  InitialCondition=0  InputProcessing=Inherited
  out0 : Outport  OutDataTypeStr=fixdt(1, 16, 10)  InitialOutput=0
  wires:
  Delay2/1 -> out0/1
  in0/1 -> Delay2/1

== system gm_combinedTxRx_AXIMM/Combined TX and RX/Receiver HDL/Frame Recover/Gardner Timing Recovery/Gardner TED Blocks/Imag Error/TED Buffer Update1/Delay3 ==
  in0 : Inport  OutDataTypeStr=fixdt(1, 16, 10)  SampleTime=1e-06
  Enable_out2 : EnablePort  OutDataTypeStr=boolean
  Delay3 : Delay  DelayLength=hex2num('3ff0000000000000')  InitialCondition=0  InputProcessing=Inherited
  out0 : Outport  OutDataTypeStr=fixdt(1, 16, 10)  InitialOutput=0
  wires:
  Delay3/1 -> out0/1
  in0/1 -> Delay3/1

== system gm_combinedTxRx_AXIMM/Combined TX and RX/Receiver HDL/Frame Recover/Gardner Timing Recovery/Gardner TED Blocks/Real Error/TED Buffer Update1/Delay ==
  in0 : Inport  OutDataTypeStr=fixdt(1, 16, 10)  SampleTime=1e-06
  Enable_out2 : EnablePort  OutDataTypeStr=boolean
  Delay : Delay  DelayLength=hex2num('3ff0000000000000')  InitialCondition=0  InputProcessing=Inherited
  out0 : Outport  OutDataTypeStr=fixdt(1, 16, 10)  InitialOutput=0
  wires:
  Delay/1 -> out0/1
  in0/1 -> Delay/1

== system gm_combinedTxRx_AXIMM/Combined TX and RX/Receiver HDL/Frame Recover/Gardner Timing Recovery/Gardner TED Blocks/Real Error/TED Buffer Update1/Delay1 ==
  in0 : Inport  OutDataTypeStr=fixdt(1, 16, 10)  SampleTime=1e-06
  Enable_out2 : EnablePort  OutDataTypeStr=boolean
  Delay1 : Delay  DelayLength=hex2num('3ff0000000000000')  InitialCondition=0  InputProcessing=Inherited
  out0 : Outport  OutDataTypeStr=fixdt(1, 16, 10)  InitialOutput=0
  wires:
  Delay1/1 -> out0/1
  in0/1 -> Delay1/1

== system gm_combinedTxRx_AXIMM/Combined TX and RX/Receiver HDL/Frame Recover/Gardner Timing Recovery/Gardner TED Blocks/Real Error/TED Buffer Update1/Delay2 ==
  in0 : Inport  OutDataTypeStr=fixdt(1, 16, 10)  SampleTime=1e-06
  Enable_out2 : EnablePort  OutDataTypeStr=boolean
  Delay2 : Delay  DelayLength=hex2num('3ff0000000000000')  InitialCondition=0  InputProcessing=Inherited
  out0 : Outport  OutDataTypeStr=fixdt(1, 16, 10)  InitialOutput=0
  wires:
  Delay2/1 -> out0/1
  in0/1 -> Delay2/1

== system gm_combinedTxRx_AXIMM/Combined TX and RX/Receiver HDL/Frame Recover/Gardner Timing Recovery/Gardner TED Blocks/Real Error/TED Buffer Update1/Delay3 ==
  in0 : Inport  OutDataTypeStr=fixdt(1, 16, 10)  SampleTime=1e-06
  Enable_out2 : EnablePort  OutDataTypeStr=boolean
  Delay3 : Delay  DelayLength=hex2num('3ff0000000000000')  InitialCondition=0  InputProcessing=Inherited
  out0 : Outport  OutDataTypeStr=fixdt(1, 16, 10)  InitialOutput=0
  wires:
  Delay3/1 -> out0/1
  in0/1 -> Delay3/1

== matlab function gm_combinedTxRx_AXIMM/Combined TX and RX/Receiver HDL/Frame Recover/Frequency Recovery/Lock Detector/MATLAB Function/RxTxFixedPointLibrary_c1_MATLAB_Function ==
  data: u input; y output
function y = abs(u)

y = fi(u,0,16,10);

== matlab function gm_combinedTxRx_AXIMM/Combined TX and RX/Receiver HDL/Viterbi Decode/Buffer/MATLAB Function1/RxTxFixedPointLibrary_c2_MATLAB_Function1 ==
  data: packetLen input; valid input; enablePop output; validOut output; crcStart input; viterbiReset output; crcOut output
function [enablePop,validOut,viterbiReset,crcOut] = manageCurrentDequeue(packetLen, valid, crcStart)

persistent currentBitsInBuffer

bitsPerCycle = uint16(2);
%bitsPerCycleDouble = uint16(4);
viterbiTracebackLengthDouble = uint16(34*2) + uint16(0);

if isempty(currentBitsInBuffer)
    currentBitsInBuffer = uint16(0);
end

if currentBitsInBuffer > viterbiTracebackLengthDouble
    currentBitsInBuffer = currentBitsInBuffer - bitsPerCycle;
    enablePop = true;
    viterbiReset = false;
    crcOut = false;
    validOut = true;
% Trigger packet at length of packet data and let Viterbi eat remaining
% data needed for traceback
elseif currentBitsInBuffer == viterbiTracebackLengthDouble
    currentBitsInBuffer = currentBitsInBuffer - bitsPerCycle;
    enablePop = true;
    viterbiReset = false;
    crcOut = true;
    validOut = false;
% Flush remaining buffered data
elseif (currentBitsInBuffer < viterbiTracebackLengthDouble) &&...
       (currentBitsInBuffer > uint16(0))
    currentBitsInBuffer = currentBitsInBuffer - bitsPerCycle;
    enablePop = true;
    viterbiReset = false;
    crcOut = false;
    validOut = false;
else
    if valid
        if crcStart
            currentBitsInBuffer = packetLen + viterbiTracebackLengthDouble + uint16(0);%bitsPerCycleDouble;
            enablePop = true;
            viterbiReset = true;
            crcOut = false;
            validOut = true;
        else
            enablePop = false;
            viterbiReset = false;
            crcOut = false;
            validOut = false;
        end
    else
        enablePop = false;
        viterbiReset = false;
        crcOut = false;     
        validOut = false;
    end
end

== matlab function gm_combinedTxRx_AXIMM/Combined TX and RX/DMA Model Driver/DMA Model Driver ==
  data: driver input; payload output; valid output boolean; enable input
function [payload,valid] = fcn(driver, enable)
%#codegen

persistent indx mode pSize

if isempty(indx)
    pSize = fi(200,0,64,0); % Size in bytes (Must be multiple of 32 bits) cannot exceed uint16 max
    indx = pSize;
    mode = int8(0);
end

setting = uint16(25*8);

if enable && driver
    valid = true;
    switch mode
        case int8(0) % Fresh packet start
            if setting>0
                pSize = fi(setting,0,64,0);
                payload = fi(setting,0,64,0);%Upper bits
                mode = int8(1);
                indx = fi(0,0,64,0);
                %new = true;
                %fprintf('(TX) Sending new packet with length: %u\n',uint64(pSize));
            else
                valid = false;
                payload = fi(0,0,64,0);
%                 new = false;
            end
        otherwise
%             new = false;
            indx = fi(indx + fi(8,0,64,0),0,64,0);
            if indx == fi(8,0,64,0)
                payload = fi(0,0,64,0);
                payload = bitset(payload,1,1);
                %                 payload = fi(uint64(12297829382473034410),0,64,0);%sum(2.^[0:2:14])); % Alternating ones and zeros
            elseif indx == pSize
                payload = fi(uint64(18446744073709551615),0,64,0); % All ones
                %                  payload = fi(uint64(12297829382473034410),0,64,0);%sum(2.^[0:2:14])); % Alternating ones and zeros
            else
                %payload = fi(uint64(randi([0 12297829382473034410])),0,64,0);%sum(2.^[0:2:14])); % Alternating ones and zeros
                payload = fi(uint64(12297829382473034410),0,64,0);%sum(2.^[0:2:14])); % Alternating ones and zeros
            end
            if indx == pSize % reached end of frame
                mode = int8(0);
            end
    end
else
    valid = false;
    payload = fi(0,0,64,0);
%     new = false;
end

== matlab function gm_combinedTxRx_AXIMM/Combined TX and RX/Transmitter HDL/Packet Generation/Payload/MATLAB Function/RxTxFixedPointLibrary_c4_MATLAB_Function ==
  data: enable input; reset output; mode output
function [reset,mode] = fcn(enable)

persistent counter

if isempty(counter)
   counter = uint8(0);
end

if enable
    counter = uint8(34*2); % tracebacklength*2
    mode = uint8(1);
    reset = true;
elseif counter>uint8(0)
    counter = counter - 1;
    mode = uint8(1);
    reset = false;
else
    mode = uint8(0);
    reset = false;
end

== matlab function gm_combinedTxRx_AXIMM/Combined TX and RX/Receiver HDL/Frame Recover/Gardner Timing Recovery/TED Lock Detector/MATLAB Function/RxTxFixedPointLibrary_c5_MATLAB_Function ==
  data: u input; y output
function y = abs(u)

y = fi(u,0,16,15);

== matlab function gm_combinedTxRx_AXIMM/Combined TX and RX/Transmitter HDL/Packet Generation/Payload/Subsystem/MATLAB Function3/RxTxFixedPointLibrary_c9_MATLAB_Function3 ==
  data: start input; enable output; done input
function enable = latch(start,done)

persistent state

if isempty(state)
   state = false; 
end

if start
    enable = true;
    state = true;
elseif done
    enable = true;
    state = false;
else
    enable = state;
end

== matlab function gm_combinedTxRx_AXIMM/Combined TX and RX/Receiver HDL/Frame Recover/Equalization and Demodulation/2 Bit Descrambler/MATLAB Function/MATLAB Function/RxTxFixedPointLibrary_c10_MATLAB_Function ==
  data: bits input; bufferA output; reset input; bufferB output
function [bufferA, bufferB] = BufferSelect(bits,reset)

persistent buffer

% Constants
initBuffer = logical([0 1 0 0 0 1 0]);

% Async
if isempty(buffer)
    buffer = initBuffer;
end

% Reset/Sync
if reset
    bufferA = initBuffer;
    bufferB = [bits(1),initBuffer(1:end-1)];
    buffer = [bits(2),bits(1),initBuffer(1:end-2)];
else
    bufferA = buffer;
    bufferB = [bits(1),buffer(1:end-1)];
    buffer = [bits(2),bits(1),buffer(1:end-2)];    
end

== matlab function gm_combinedTxRx_AXIMM/Combined TX and RX/Receiver HDL/CRC Check and DMA Pack/DMA Interface/Bit Packer/RxTxFixedPointLibrary_c11_Bit_Packer ==
  data: bitIn input; byteOut output; startIn input; endIn input; err input; validIn input; validOut output; startOut output
function [byteOut,validOut,startOut] = BitPacker(bitIn, startIn, endIn, err, validIn)

% This block will pack bits into bytes with start boundaries


% Constants
bits2Pack = uint8(64); % byteReg must contain this many bits
zero64 = fi(0,0,64,0);
% NOTE: Frames but be a multiple of bits2Pack or bits will be trimmed from
% end

persistent byteReg byteIndx setStartFlag

if isempty(byteIndx)
    byteReg  = fi(0,0,64,0);
    byteIndx = uint8(1);
    setStartFlag = false;
end

if validIn
    if startIn % Reset
        byteReg = bitset(zero64,1,bitIn);
        byteIndx = uint8(2);
        validOut = false;
        setStartFlag = true;
        startOut = false;
    else
        byteReg = bitset(byteReg,byteIndx,bitIn);
        if byteIndx >= bits2Pack
            byteIndx = uint8(1);
            validOut = true;
            startOut = setStartFlag;
            setStartFlag = false;
        else
            byteIndx = byteIndx + uint8(1);
            validOut = false;
            startOut = false;
        end
    end
elseif endIn % Append error bit to last byte
    byteReg = fi(err,0,64,0);
    validOut = true;
    startOut = false;
else
    validOut = false;
    startOut = false;
end

byteOut = byteReg;

== matlab function gm_combinedTxRx_AXIMM/Combined TX and RX/Receiver HDL/Frame Recover/Enable Equalizer and Packet Decode (Latch)/RxTxFixedPointLibrary_c12_Enable_Equalizer_and_Packet_Decode__L ==
  data: start input; enable output; validIn input
function enable = Counter(start,validIn)

persistent count maxCount lastEOF

if isempty(count)
    count = uint32(0);
    maxCount = uint32(2^16); % Largest possible packet length
    lastEOF = false;
end

eof = false;

if validIn
    % Got a barker preamble start allowing data into equalizer
    if start
        count = maxCount;
    end
    
    % Check on change from true to false
    if lastEOF && ~eof
        %     fprintf('Frame end reached\n');
        count = uint32(0);
    end
    lastEOF = eof;
    
    % Past end of max frame size
    if count>0
        count = count - uint32(1);
    end
    
    % Enable downstream
    enable = count>uint32(0);
else
    enable = false;
end

== matlab function gm_combinedTxRx_AXIMM/Combined TX and RX/Receiver HDL/Frame Recover/Equalization and Demodulation/Header Controller/Header Controller/RxTxFixedPointLibrary_c15_Header_Controller ==
  data: enableDownstream output; headerStart input; packetLenBitsOut output; data input; resetViterbi output; crcStart output; status output; s1 output; s2 output
function [enableDownstream,packetLenBitsOut,resetViterbi,crcStart,status,s1,s2] = EvalHeader(headerStart, data)

persistent counter sum1 sum2 packetLenBits lastMode savedPacketLenBits

% The header contains 16 bits, but each bit is duplicated to make checking
% easier
%
% Note this block works on symbols (2bits) but 1 symbol -> 1 decoded bit
%
% PacketLength = (Data+CRC+40(TB)+68)/CodeRate
%
% NOTE TAIL BITS HERE ARE REALLY USED TO DEAL WITH VITERBI LAG SO:
% TailBitsWithLagPadding > TracebackLength

%% Constants
numHeaderBits = uint8(16); % Header is this many bits
powersOfTwo = uint32([1 2 4 8 16 32 64 128 256 512 1024 2048 4096 8192 16384 32768]);
CodeRateINV = uint32(2);%1/CodeRate;
TailBitsWithLagPadding = uint32(uint32(40)+34*2+1); % was +1
% Flag when CRC porition of packet starts relative to header
crcSignalStartLocation = uint32((TailBitsWithLagPadding)*CodeRateINV); % Must be even

% Async
if isempty(counter)
    packetLenBits = uint32(0);
    sum1 = uint32(0);
    sum2 = uint32(0);
    counter = uint8(numHeaderBits);
    lastMode = uint8(3);
    savedPacketLenBits = uint16(0);
end


%% Sync
% Got a header now enable certain mode
if headerStart
    mode = uint8(0);
else
    mode = lastMode;
end

switch mode
    %% Reset on preamble flag and setup for header processing
    case uint8(0)
        crcStart = false;
        resetViterbi = false;
        enableDownstream = false;
        sum1 = uint32(0);
        sum2 = uint32(0);
        counter = uint8(1);
        lastMode = uint8(1); % Go to next state
        packetLenBitsOut = uint16(0);
        status = uint8(0); s1 = uint32(0); s2 = uint32(0);
        
    %% Process header
    case 1 
        crcStart = false;
        enableDownstream = false;
        
        % Convert header bits (bit by bit)
        if data(1)
            sum1 = sum1 + powersOfTwo(counter);
        end
        if data(2)
            sum2 = sum2 + powersOfTwo(counter);
        end
        counter = counter + uint8(1);
        
        if counter>numHeaderBits
            % Check header
            if sum1~=sum2 % Fail
                packetLenBits = uint32(0);
                lastMode = uint8(3);
                resetViterbi = false;
                packetLenBitsOut = uint16(0);
                savedPacketLenBits = uint16(0);
                status = uint8(2); s1 = sum1; s2 = sum2;
            else % Pass
                % Saved header info and trigger downstream
                packetLenBits = uint32(sum1);
                lastMode = uint8(2);
                resetViterbi = true;
                packetLenBitsOut = uint16(sum1-crcSignalStartLocation);
                savedPacketLenBits = uint16(sum1-crcSignalStartLocation);
                status = uint8(1); s1 = sum1; s2 = sum2;
            end
        else
            status = uint8(0); s1 = uint32(0); s2 = uint32(0);
            packetLenBitsOut = uint16(0);
            resetViterbi = false;
        end
        
    %% Decrement sample counter
    case 2 
        status = uint8(0); s1 = uint32(0); s2 = uint32(0);
        resetViterbi = false;
        crcStart = (packetLenBits==crcSignalStartLocation);
        if packetLenBits>uint32(0)
            enableDownstream = true;
            packetLenBits = packetLenBits - uint32(2); % We get 2 bits each call
            packetLenBitsOut = savedPacketLenBits;
        else
            enableDownstream = false;
            lastMode = uint8(3);
            packetLenBitsOut = uint16(0); %Reset
            savedPacketLenBits = uint16(0);%Reset
        end
            
    %% Not processing anything
    otherwise % mode>2
        status = uint8(0); s1 = uint32(0); s2 = uint32(0);
        crcStart = false;
        resetViterbi = false;
        enableDownstream = false;
        packetLenBitsOut = uint16(0);
end

== matlab function gm_combinedTxRx_AXIMM/Combined TX and RX/Receiver HDL/Frame Recover/Frequency Recovery/PED/RxTxFixedPointLibrary_c16_PED ==
  data: In input; e output
function e  = PED(In)

OP2 = real(In);
OP1 = imag(In);

Real = OP2;
Imag = OP1;

if (bitget(Real,16)==true) % real component is negative
    OP1 = fi(-Imag,1,16,13);
end
if (bitget(Imag,16)==true) % imaginary component is negative
    OP2 = fi(-Real,1,16,13);
end

e= fi(OP1-OP2,1,16,10);

%e = sign(real(In)).*imag(In) - sign(imag(In)).*real(In);
